simulink model "dmc_ut"  (Simulink 8.1)
settings: Solver=ode1  StartTime=0.0  StopTime=Inf  FixedStep=0.001  RelTol=1e-3
PostLoadFcn:
  | , if any(exist('dsrtsu_mdlpostloadfcn', 'file') == [2, 3, 6]), try dsrtsu_mdlpostloadfcn('Execute', bdroot); catch fprintf('Error in PostLoadFcn (dsrtsu_mdlpostloadfcn) for model "%s":\n %s\n', bdroot, lasterr); end, end,
libraries: siltestlib x4, afa x1, hcu_lib x1
settings Model: DSRTSU_INTERNAL_RTI_VER=450  DSRTSU_INTERNAL_RTI_TYPE=rti1401  RTICANMMDATA=struct('GeneralSetupData',struct('modelroot','D:\Soichi\SVNDATA\IDIADA_ADAS\trunk\AdasDragon\software\sw_development\arch\app\fcw','generalsettings',struct('filesettings',struct('destfolder',struct('Name','RTICANMM_FILES','Check',1),'buildfolder',struct('Name','.','Check',1),'AbsDestfolder',struct('Name','D:\Soichi\SVNDATA\IDIADA_ADAS\trunk\AdasDragon\software\sw_development\arch\app\fcw\RTICANMM_FILES'),'AbsBuildfolder',struct('Name','D:\Soichi\SVNDATA\IDIADA_ADAS\trunk\AdasDragon\software\sw_development\arch\app\fcw'))),'options',struct('addpaths',1,'rmpaths',1,'addtrcexclusion',logical(1),'cannavigator',struct('checkmonitoring',0),'show_usrtrc',0,'use_usrtrc',0),'advanced',struct('options',[1 1 1 1 1 1 1 1 1 1 1 1 1 1 1 1 1 1 1 1 1 1 1 1 1 1 1 1 1 1 1 1 1 1 1 1 1 1 1 1 1 1 1 1 1 1 1 1 1 1 1 1 1 1 1 1 1 1 1 1 1 1 1 1 1 1 1 1 1 1 1 1 1 1 1 1 1 1 1 1 1 1 1 1 1 1 1 1 1 1 1 1 1 1 1 1 1 1 1 1]),'MPSetup',{{}},'modelname','dmc_ut','block','dmc_ut'))  DSRTSU_INTERNAL_RTIFPGA=40  Creator=tescamilla  LastModifiedBy=AT015411  BufferReuse=off
settings DataIOCC: SignalLoggingSaveFormat=Dataset
settings OptimizationCC: BlockReduction=off  OptimizeBlockIOStorage=off  BufferReuse=off  ExpressionFolding=off  ExpressionDepthLimit=128  LocalBlockOutputs=off
settings DebuggingCC: FcnCallInpInsideContextMsg=EnableAllAsError
settings HardwareCC: ProdIntDivRoundTo=Zero  ProdEndianess=BigEndian  ProdHWDeviceType=Generic->Custom  TargetIntDivRoundTo=Zero  TargetEndianess=BigEndian  TargetHWDeviceType=Generic->Custom
settings RTWCC: SystemTargetFile=rti1401.tlc  MakeCommand=make_rti  TemplateMakefile=rti1401.tmf  Description=dSPACE DS1401 Hardware Platform  ProcessScript=rti1401_make_rtw_hook
settings STFCustomTargetCC: CodeReplacementLibrary=ANSI_C  ParMdlRefBuildCompliant=on  GeneratePreprocessorConditionals=Disable all  MatFileLogging=on  SystemTargetFile=rti1401.tlc
settings GRTTargetCC: CompOptLevelCompliant=off  ConcurrentExecutionCompliant=off  ExtModeMexFile=noextcomm
settings CustomProperty: DataType=RTWOptions_EnumType_D__Program Files_dSPACE RCPHIL 2014-B_MATLAB_RTI_RTI1401_TLC_rti1401_1InitialSimState  Value=RUN
settings EnumStrPairs: String=RUN

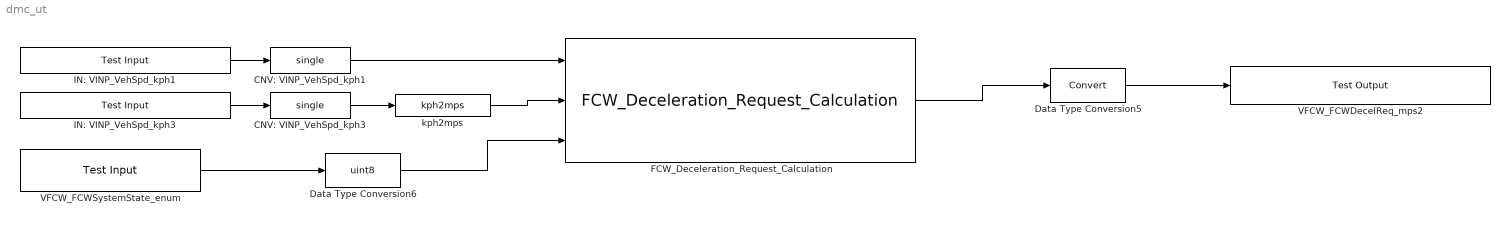
== system dmc_ut ==
  CNV: VINP_VehSpd_kph1 : DataTypeConversion  OutDataTypeStr=single
  CNV: VINP_VehSpd_kph3 : DataTypeConversion  OutDataTypeStr=single
  Data Type Conversion5 : DataTypeConversion
  Data Type Conversion6 : DataTypeConversion  OutDataTypeStr=uint8
  FCW_Deceleration_Request_Calculation : afa/Actions_for_FCW_Acting/FCW_Deceleration_Request_Calculation
  IN: VINP_VehSpd_kph1 : siltestlib/Test Input  varname=VIFO_FCWTargetVehicleTtcX_ms  sampletime=-1
  IN: VINP_VehSpd_kph3 : siltestlib/Test Input  varname=VIFO_FCWTargetVehRelSpeed_kph  sampletime=-1
  VFCW_FCWDecelReq_mps2 : siltestlib/Test Output  varname=VFCW_FCWDecelReq_mps2  sampletime=-1
  VFCW_FCWSystemState_enum : siltestlib/Test Input  varname=VFCW_FCWSystemState_enum  sampletime=-1
  kph2mps : hcu_lib/kph2mps
  wires:
  CNV: VINP_VehSpd_kph1/1 -> FCW_Deceleration_Request_Calculation/1
  CNV: VINP_VehSpd_kph3/1 -> kph2mps/1
  IN: VINP_VehSpd_kph3/1 -> CNV: VINP_VehSpd_kph3/1
  IN: VINP_VehSpd_kph1/1 -> CNV: VINP_VehSpd_kph1/1
  kph2mps/1 -> FCW_Deceleration_Request_Calculation/2
  FCW_Deceleration_Request_Calculation/1 -> Data Type Conversion5/1
  Data Type Conversion5/1 -> VFCW_FCWDecelReq_mps2/1
  VFCW_FCWSystemState_enum/1 -> Data Type Conversion6/1
  Data Type Conversion6/1 -> FCW_Deceleration_Request_Calculation/3
